simulink model "heli_q8_3_542"  (R2014a)
settings: Solver=ode1  StartTime=0.0  StopTime=inf  FixedStep=0.002  RelTol=1e-3
PostLoadFcn:
  | qc_set_target_type(getConfigSet(bdroot, 'QUARC Default Target Configuration'));
values from neighbouring files (symbols this model uses):
  A_L = [0 1 0 0 0 0; 0 0 0 0 0 0; 0 0 0 1 0 0; 0 0 0 0 0 0; 0 0 0 0 0 1; K_3 0 0 0 0 0]    [init_heli.m]
  B_L = transpose(place(transpose(A_L),transpose(C_B_L),p_B))    [init_heli.m]
  C_L = [1 0 0 0 0 0; 0 0 1 0 0 0; 0 0 0 0 1 0]    [init_heli.m]
  Joystick_gain_x = 1.5    [init_heli.m]
  Joystick_gain_y = -1.5    [init_heli.m]
  K_L = lqr(A_PI,B_PI,Q_L,R_L)    [init_heli.m]
  L = transpose(place(transpose(A_L),transpose(C_L),p))    [init_heli.m]
  P_L = inv(C*inv(B*K_P_L-A)*B)    [init_heli.m]
  V_s_star = 6.5    [init_heli.m]
undefined symbols (not defined in the file or in its folder): HIL, qc_get_step_size
libraries: simulink_extras x6, quarc_library x4
settings Model: SimulationMode=external  ExtModeTrigDuration=500000  Creator=Rchan  LastModifiedBy=mekvamme
settings SolverCC: PositivePriorityOrder=on
settings DataIOCC: LimitDataPoints=off  MaxDataPoints=10000  SignalLoggingSaveFormat=ModelDataLogs
settings OptimizationCC: ExpressionDepthLimit=2147483647  InitFltsAndDblsToZero=on
settings DebuggingCC: SaveWithParameterizedLinksMsg=none  UnderspecifiedInitializationDetection=Classic  MultiTaskDSMMsg=warning  MultiTaskCondExecSysMsg=none  FcnCallInpInsideContextMsg=UseLocalSettings  StateNameClashWarn=warning
settings RTWCC: SystemTargetFile=quarc_win64.tlc  TemplateMakefile=quarc_default_tmf  Description=QUARC Win64 Target  ProcessScript=quarc_win64_make_rtw_hook
settings STFCustomTargetCC: CPPClassGenCompliant=on
settings GRTTargetCC: ParMdlRefBuildCompliant=off  CompOptLevelCompliant=off  CombineOutputUpdateFcns=off  MatFileLogging=off  GRTInterface=on  ExtMode=on  ExtModeMexFile=quarc_comm

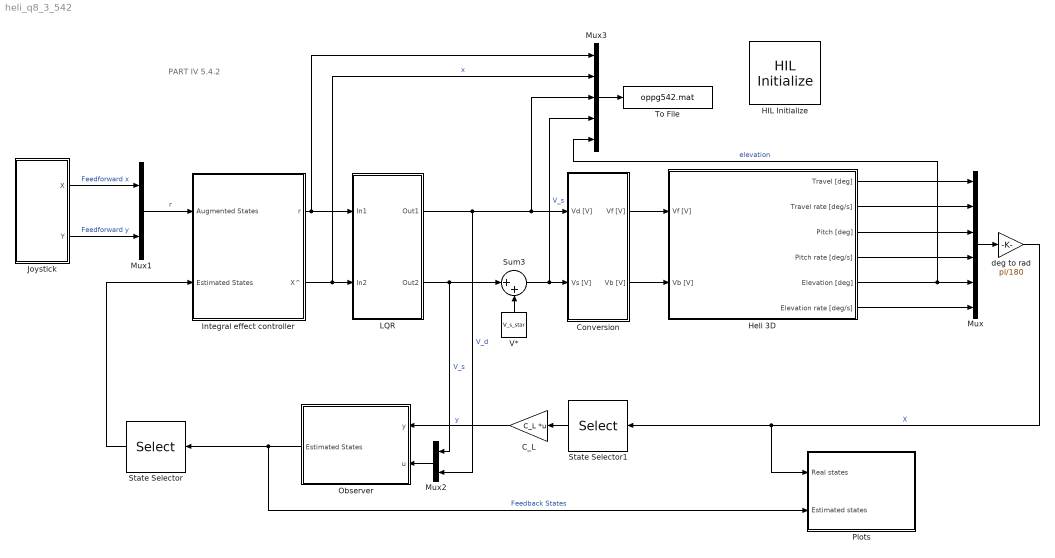
== system heli_q8_3_542 ==
  note: PART IV
      | 5.4.2
  C_L : Gain  Gain=C_L  Multiplication=Matrix(K*u) (u vector)
  Conversion : Subsystem
  HIL Initialize : quarc_library/Data Acquisition/Generic/Configuration/HIL Initialize  Priority=-99  object_name=HIL-1  board_type=q8_usb  board_number=0  board_options=update_rate=normal;decimation=1  exclusive=off  active=off  hardware_clocks=[0:2]  clock_modes=[]  initial_clock_frequencies=[]  set_clock_params_at_start=off  set_clock_params_at_switch_in=off  set_clock_frequencies_at_start=off  set_clock_frequencies_at_switch_in=off  analog_input_channels=[0:7]  analog_input_maximums=10  analog_input_minimums=-10  set_analog_input_params_at_start=on  set_analog_input_params_at_switch_in=off  analog_output_channels=[0:7]  analog_output_maximums=10  analog_output_minimums=-10  initial_analog_outputs=[0]  final_analog_outputs=[0]  watchdog_analog_outputs=0  set_analog_output_params_at_start=on  set_analog_output_params_at_switch_in=off  set_analog_outputs_at_start=on  set_analog_outputs_at_switch_in=off  set_analog_outputs_at_terminate=on  set_analog_outputs_at_switch_out=off  set_analog_outputs_on_watchdog=off  digital_input_channels=[]  digital_output_channels=[]  digital_output_configuration=[]  initial_digital_outputs=[1]  final_digital_outputs=[1]  watchdog_digital_outputs=[1]  set_digital_output_params_at_start=off  set_digital_output_params_at_switch_in=off  set_digital_outputs_at_start=on  set_digital_outputs_at_switch_in=off  set_digital_outputs_at_terminate=on  set_digital_outputs_at_switch_out=off  set_digital_outputs_on_watchdog=off  encoder_channels=[0:7]  quadrature=[4]  encoder_filter_frequency=[]  initial_encoder_counts=[0]  set_encoder_params_at_start=on  set_encoder_params_at_switch_in=off  set_encoder_counts_at_start=on  set_encoder_counts_at_switch_in=off  pwm_channels=[0:7]  pwm_modes=0  pwm_frequency=99.532799999999995e6/4095  pwm_configuration=[0]  pwm_alignment=[0]  pwm_polarity=[1]  pwm_leading_deadband=[0]  pwm_trailing_deadband=[0]  initial_pwm_outputs=[0]  final_pwm_outputs=[0]  watchdog_pwm_outputs=[0]  set_pwm_params_at_start=on  set_pwm_params_at_switch_in=off  set_pwm_outputs_at_start=on  set_pwm_outputs_at_switch_in=off  set_pwm_outputs_at_terminate=on  set_pwm_outputs_at_switch_out=off  set_pwm_outputs_on_watchdog=off  other_output_channels=[]  initial_other_outputs=[]  final_other_outputs=[]  watchdog_other_outputs=[]  set_other_outputs_at_start=off  set_other_outputs_at_switch_in=off  set_other_outputs_at_terminate=off  set_other_outputs_at_switch_out=off  set_other_outputs_on_watchdog=off
  Heli 3D : Subsystem
  Integral effect controller : Subsystem
  Joystick : Subsystem
  LQR : Subsystem
  Mux : Mux  Inputs=6
  Mux1 : Mux  Inputs=2
  Mux2 : Mux  Inputs=2
  Mux3 : Mux  Inputs=5
  Observer : Subsystem
  Plots : Subsystem
  State Selector : Selector  InputPortWidth=6  Indices=[1 2 4]
  State Selector1 : Selector  InputPortWidth=6  Indices=[3 4 5 6 1 2]
  Sum3 : Sum  Inputs=|++
  To File : ToFile  RequirementInfo={'linktype_rmi_matlab' 'save.mat' '@save' 'true' 'save' '' } %GIDa_040f6fd3_b98c_4d05_89a6_2c52f44394e1  Filename=oppg542.mat  MatrixName=var
  V* : Constant  Value=V_s_star
  deg to rad : Gain  Gain=pi/180
  wires:
  Conversion/2(Vb [V]) -> Heli 3D/2(Vb [V])
  Conversion/1(Vf [V]) -> Heli 3D/1(Vf [V])
  Heli 3D/1(Travel [deg]) -> Mux/1
  Heli 3D/2(Travel rate [deg/s]) -> Mux/2
  Heli 3D/4(Pitch rate [deg/s]) -> Mux/4
  Heli 3D/6(Elevation rate [deg/s]) -> Mux/6
  Mux/1 -> deg to rad/1
  Heli 3D/3(Pitch [deg]) -> Mux/3
  Sum3/1 -> Conversion/2(Vs [V]), Mux3/4  "V_s"
  V*/1 -> Sum3/2
  Mux3/1 -> To File/1
  LQR/1(Out1) -> Conversion/1(Vd [V]), Mux3/3, Mux2/2  "V_d"
  Integral effect controller/2(X^) -> Mux3/2, LQR/2(In2)  "x"
  Mux1/1 -> Integral effect controller/1(Augmented States)  "r"
  C_L/1 -> Observer/1(y)  "y"
  deg to rad/1 -> Plots/1(Real states), State Selector1/1  "X"
  State Selector/1 -> Integral effect controller/2(Estimated States)
  Integral effect controller/1(r) -> Mux3/1, LQR/1(In1)
  Heli 3D/5(Elevation [deg]) -> Mux3/5, Mux/5  "elevation"
  Joystick/1(X) -> Mux1/1  "Feedforward x"
  Joystick/2(Y) -> Mux1/2  "Feedforward y"
  State Selector1/1 -> C_L/1
  Mux2/1 -> Observer/2(u)
  Observer/1(Estimated States) -> Plots/2(Estimated states), State Selector/1  "Feedback States"
  LQR/2(Out2) -> Mux2/1, Sum3/1  "V_s"

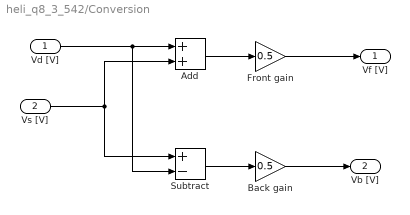
== system heli_q8_3_542/Conversion ==
  Vd [V] : Inport
  Vs [V] : Inport  Port=2
  Add : Sum
  Back gain : Gain  Gain=0.5
  Front gain : Gain  Gain=0.5
  Subtract : Sum  Inputs=+-
  Vf [V] : Outport
  Vb [V] : Outport  Port=2
  wires:
  Vd [V]/1 -> Subtract/2, Add/1
  Vs [V]/1 -> Subtract/1, Add/2
  Subtract/1 -> Back gain/1
  Back gain/1 -> Vb [V]/1
  Add/1 -> Front gain/1
  Front gain/1 -> Vf [V]/1

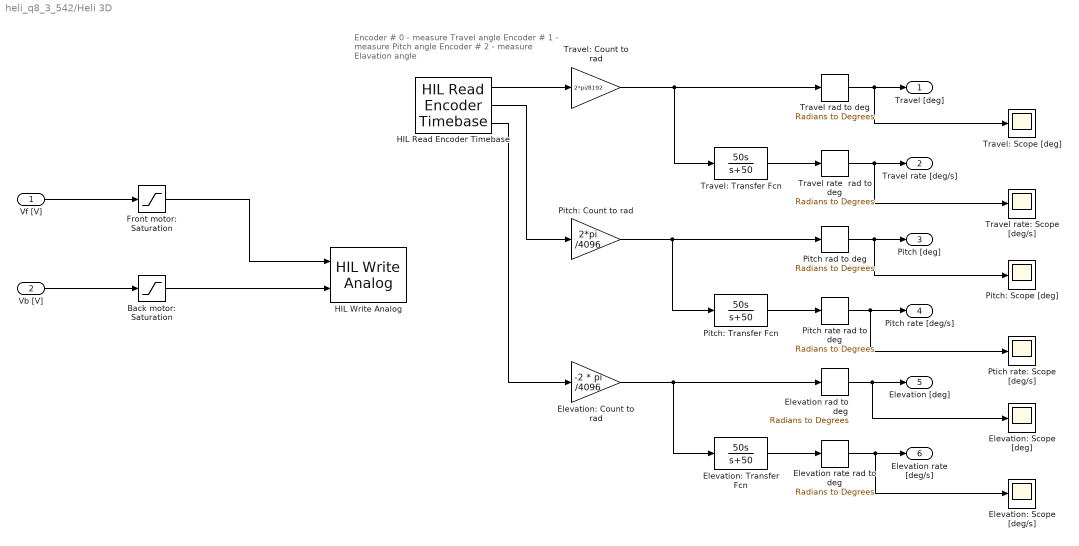
== system heli_q8_3_542/Heli 3D ==
  note: Encoder # 0 - measure Travel angle
      | Encoder # 1 - measure Pitch angle
      | Encoder # 2 - measure Elavation angle
  Vf [V] : Inport
  Vb [V] : Inport  Port=2
  Back motor: Saturation : Saturate  UpperLimit=5  LowerLimit=-5
  Elevation rad to deg : simulink_extras/Transformations/Radians to Degrees
  Elevation rate rad to deg : simulink_extras/Transformations/Radians to Degrees
  Elevation: Count to rad : Gain  Gain=-2 * pi /4096
  Elevation: Scope [deg/s] : Scope
      settings: YMin=-15  YMax=15  SaveName=ScopeData13
  Elevation: Scope [deg] : Scope
      settings: TimeRange=10  YMin=-0  YMax=30  SaveName=ScopeData12
  Elevation: Transfer Fcn : TransferFcn  Numerator=[50 0]  Denominator=[1 50]
  Front motor: Saturation : Saturate  UpperLimit=5  LowerLimit=-5
  HIL Read Encoder Timebase : quarc_library/Data Acquisition/Generic/Timebases/HIL Read Encoder Timebase  object_name=HIL-1  clock=0  channels=[0:2]  samples_in_buffer=max(ceil(1/qc_get_step_size), 1)  active=on  vector_output=off  data_type_mode=Inherit via back propagation  data_type=double
  HIL Write Analog : quarc_library/Data Acquisition/Generic/Immediate I//O/HIL Write Analog  object_name=HIL-1  channels=[0:1]  sample_time=-1  active=off  vector_input=off
  Pitch rad to deg : simulink_extras/Transformations/Radians to Degrees
  Pitch rate rad to deg : simulink_extras/Transformations/Radians to Degrees
  Pitch: Count to rad : Gain  Gain=2*pi /4096
  Pitch: Scope [deg] : Scope
      settings: ShowLegends=on  YMin=-45  YMax=55  SaveName=ScopeData10
  Pitch: Transfer Fcn : TransferFcn  Numerator=[50 0]  Denominator=[1 50]
  Ptich rate: Scope [deg/s] : Scope
      settings: YMin=-15  YMax=15  SaveName=ScopeData11
  Travel rad to deg : simulink_extras/Transformations/Radians to Degrees
  Travel rate  rad to deg : simulink_extras/Transformations/Radians to Degrees
  Travel rate: Scope [deg/s] : Scope
      settings: YMin=-35  YMax=25  SaveName=ScopeData9
  Travel: Count to rad : Gain  Gain=2*pi/8192
  Travel: Scope [deg] : Scope
      settings: YMin=-30  YMax=130  SaveName=ScopeData8
  Travel: Transfer Fcn : TransferFcn  Numerator=[50 0]  Denominator=[1 50]
  Travel [deg] : Outport
  Travel rate [deg/s] : Outport  Port=2
  Pitch [deg] : Outport  Port=3
  Pitch rate [deg/s] : Outport  Port=4
  Elevation [deg] : Outport  Port=5
  Elevation rate [deg/s] : Outport  Port=6
  wires:
  HIL Read Encoder Timebase/1 -> Travel: Count to rad/1
  HIL Read Encoder Timebase/2 -> Pitch: Count to rad/1
  HIL Read Encoder Timebase/3 -> Elevation: Count to rad/1
  Travel: Count to rad/1 -> Travel: Transfer Fcn/1, Travel rad to deg/1
  Travel: Transfer Fcn/1 -> Travel rate  rad to deg/1
  Pitch: Count to rad/1 -> Pitch: Transfer Fcn/1, Pitch rad to deg/1
  Pitch: Transfer Fcn/1 -> Pitch rate rad to deg/1
  Elevation: Count to rad/1 -> Elevation: Transfer Fcn/1, Elevation rad to deg/1
  Elevation: Transfer Fcn/1 -> Elevation rate rad to deg/1
  Travel rad to deg/1 -> Travel: Scope [deg]/1, Travel [deg]/1
  Travel rate  rad to deg/1 -> Travel rate: Scope [deg/s]/1, Travel rate [deg/s]/1
  Pitch rad to deg/1 -> Pitch: Scope [deg]/1, Pitch [deg]/1
  Pitch rate rad to deg/1 -> Ptich rate: Scope [deg/s]/1, Pitch rate [deg/s]/1
  Elevation rad to deg/1 -> Elevation: Scope [deg]/1, Elevation [deg]/1
  Elevation rate rad to deg/1 -> Elevation: Scope [deg/s]/1, Elevation rate [deg/s]/1
  Vf [V]/1 -> Front motor: Saturation/1
  Vb [V]/1 -> Back motor: Saturation/1
  Front motor: Saturation/1 -> HIL Write Analog/1
  Back motor: Saturation/1 -> HIL Write Analog/2

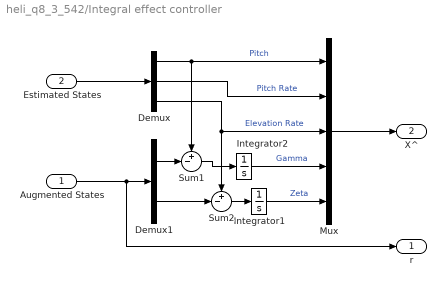
== system heli_q8_3_542/Integral effect controller ==
  Augmented States : Inport
  Estimated States : Inport  Port=2
  " Integrator2" : Integrator
  Demux : Demux  Outputs=3
  Demux1 : Demux  Outputs=2
  Integrator1 : Integrator
  Mux : Mux  Inputs=5
  Sum1 : Sum  Inputs=+-|
  Sum2 : Sum  Inputs=+-|
  r : Outport  InitialOutput=0
  X^ : Outport  Port=2  InitialOutput=0
  wires:
  Mux/1 -> X^/1
  Demux/2 -> Mux/2  "Pitch Rate"
  Demux/1 -> Mux/1, Sum1/1  "Pitch"
  Demux/3 -> Sum2/1, Mux/3  "Elevation Rate"
  Demux1/1 -> Sum1/2
  Demux1/2 -> Sum2/2
  Sum1/1 -> " Integrator2"/1
  Sum2/1 -> Integrator1/1
  " Integrator2"/1 -> Mux/4  "Gamma"
  Integrator1/1 -> Mux/5  "Zeta"
  Augmented States/1 -> r/1, Demux1/1
  Estimated States/1 -> Demux/1

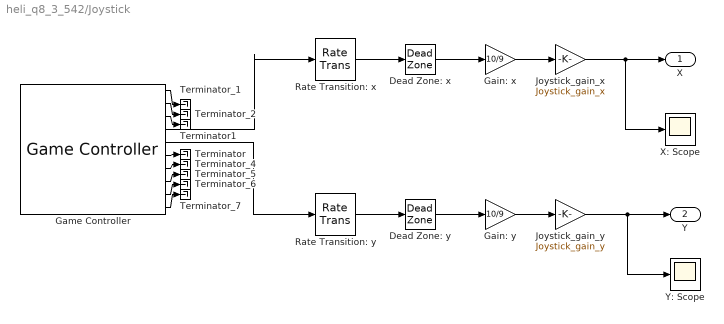
== system heli_q8_3_542/Joystick ==
  Dead Zone: x : DeadZone  LowerValue=-0.1  UpperValue=0.1  SaturateOnIntegerOverflow=on
  Dead Zone: y : DeadZone  LowerValue=-0.1  UpperValue=0.1  SaturateOnIntegerOverflow=on
  Gain: x : Gain  Gain=10/9
  Gain: y : Gain  Gain=10/9
  Game Controller : quarc_library/Devices/Peripherals/Target/Game Controller  controller=1  buffer_size=12  deadzone=[]  saturation=[]  sample_time=max(qc_get_step_size, 0.01)  auto_center=off  enabled=on
  Joystick_gain_x : Gain  Gain=Joystick_gain_x
  Joystick_gain_y : Gain  Gain=Joystick_gain_y
  Rate Transition: x : RateTransition
  Rate Transition: y : RateTransition
  Terminator : Terminator
  Terminator1 : Terminator
  Terminator_{1..2,4..7} (6 alike) : Terminator
  X: Scope : Scope
      settings: YMin=-1  YMax=1  SaveName=ScopeData7
  Y: Scope : Scope
      settings: YMin=-10  YMax=10  SaveName=ScopeData5
  X : Outport
  Y : Outport  Port=2
  wires:
  Rate Transition: y/1 -> Dead Zone: y/1
  Rate Transition: x/1 -> Dead Zone: x/1
  Game Controller/5 -> Rate Transition: y/1
  Game Controller/4 -> Rate Transition: x/1
  Game Controller/1 -> Terminator_1/1
  Game Controller/2 -> Terminator_2/1
  Game Controller/7 -> Terminator_4/1
  Game Controller/8 -> Terminator_5/1
  Game Controller/9 -> Terminator_6/1
  Game Controller/10 -> Terminator_7/1
  Game Controller/3 -> Terminator1/1
  Game Controller/6 -> Terminator/1
  Dead Zone: x/1 -> Gain: x/1
  Dead Zone: y/1 -> Gain: y/1
  Gain: x/1 -> Joystick_gain_x/1
  Gain: y/1 -> Joystick_gain_y/1
  Joystick_gain_x/1 -> X/1, X: Scope/1
  Joystick_gain_y/1 -> Y: Scope/1, Y/1

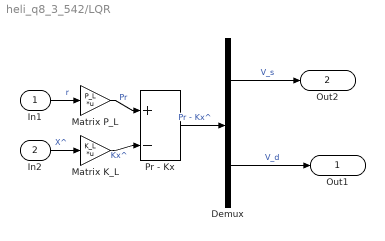
== system heli_q8_3_542/LQR ==
  In1 : Inport
  In2 : Inport  Port=2
  Demux : Demux  Outputs=2
  Matrix K_L : Gain  Gain=K_L  Multiplication=Matrix(K*u)
  Matrix P_L : Gain  Gain=P_L  Multiplication=Matrix(K*u)
  Pr - Kx : Sum  Inputs=+|-
  Out1 : Outport
  Out2 : Outport  Port=2
  wires:
  In1/1 -> Matrix P_L/1  "r"
  In2/1 -> Matrix K_L/1  "X^"
  Matrix K_L/1 -> Pr - Kx/2  "Kx^"
  Matrix P_L/1 -> Pr - Kx/1  "Pr"
  Pr - Kx/1 -> Demux/1  "Pr - Kx^"
  Demux/1 -> Out2/1  "V_s"
  Demux/2 -> Out1/1  "V_d"

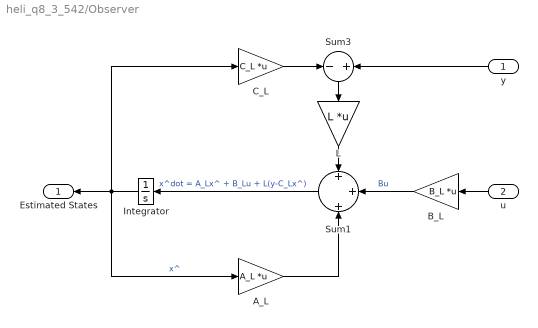
== system heli_q8_3_542/Observer ==
  y : Inport
  u : Inport  Port=2
  A_L : Gain  Gain=A_L  Multiplication=Matrix(K*u) (u vector)
  B_L : Gain  Gain=B_L  Multiplication=Matrix(K*u) (u vector)
  C_L : Gain  Gain=C_L  Multiplication=Matrix(K*u) (u vector)
  Integrator : Integrator
  L : Gain  Gain=L  Multiplication=Matrix(K*u) (u vector)
  Sum1 : Sum  Inputs=+|+|+
  Sum3 : Sum  Inputs=-|+
  Estimated States : Outport  InitialOutput=0
  wires:
  Integrator/1 -> Estimated States/1, C_L/1, A_L/1  "x^"
  y/1 -> Sum3/2
  Sum3/1 -> L/1
  L/1 -> Sum1/1
  u/1 -> B_L/1
  Sum1/1 -> Integrator/1  "x^dot = A_Lx^ + B_Lu + L(y-C_Lx^)"
  C_L/1 -> Sum3/1
  A_L/1 -> Sum1/3
  B_L/1 -> Sum1/2  "Bu"

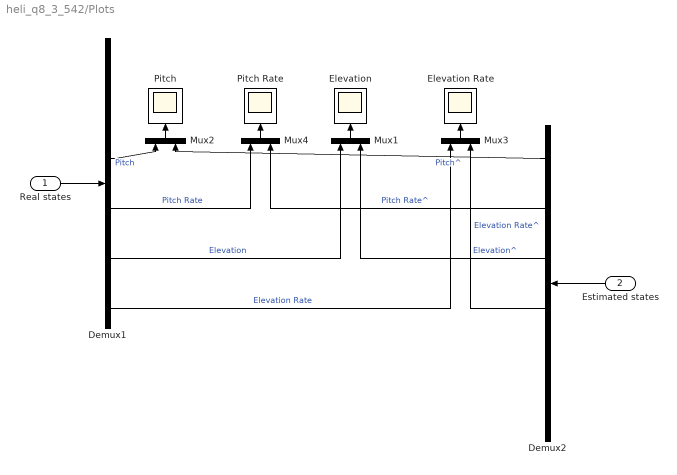
== system heli_q8_3_542/Plots ==
  Real states : Inport
  Estimated states : Inport  Port=2
  Demux1 : Demux  Outputs=6
  Demux2 : Demux  Outputs=6
  Elevation : Scope
      settings: ShowLegends=on  SaveName=ScopeData3
  Elevation Rate : Scope
      settings: ShowLegends=on  SaveName=ScopeData4
  Mux{1..4} (4 alike) : Mux  Inputs=2
  Pitch : Scope
      settings: ShowLegends=on
  Pitch Rate : Scope
      settings: ShowLegends=on
  wires:
  Real states/1 -> Demux1/1
  Estimated states/1 -> Demux2/1
  Demux2/1 -> Mux2/2  "Pitch^"
  Demux2/2 -> Mux4/2  "Pitch Rate^"
  Demux2/3 -> Mux1/2  "Elevation^"
  Demux2/4 -> Mux3/2  "Elevation Rate^"
  Demux1/3 -> Mux2/1  "Pitch"
  Demux1/4 -> Mux4/1  "Pitch Rate"
  Demux1/5 -> Mux1/1  "Elevation"
  Demux1/6 -> Mux3/1  "Elevation Rate"
  Mux2/1 -> Pitch/1
  Mux4/1 -> Pitch Rate/1
  Mux1/1 -> Elevation/1
  Mux3/1 -> Elevation Rate/1
